simulink model "pole_cart_model"  (R2019b)
settings: Solver=VariableStepAuto  StartTime=0.0  StopTime=5  RelTol=1e-3
values from neighbouring files (symbols this model uses):
  K = zeros(Nu, Nx, Nt-1)    [run_ilqr.m]    (also in run_model.m = [ -70.7107  -37.8345  105.5298   20.9238])
  x0 = [0; 0; 0; 0]    [run_ilqr.m]    (also in run_model.m = [0;0;0;0])
settings Model: Creator=bbamin  LastModifiedBy=bbamin

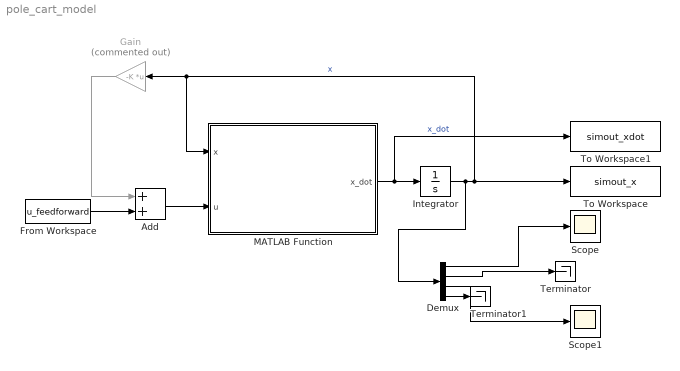
== system pole_cart_model ==
  Add : Sum
  Demux : Demux
  From Workspace : FromWorkspace  VariableName=u_feedforward  SampleTime=0  Interpolate=off  OutputAfterFinalValue=Setting to zero
  Gain : Gain  Commented=on  Gain=-K  Multiplication=Matrix(K*u)
  Integrator : Integrator  InitialCondition=x0
  MATLAB Function : MATLAB Function  TreatAsAtomicUnit=on
  Scope : Scope
  Scope1 : Scope
  Terminator : Terminator
  Terminator1 : Terminator
  To Workspace : ToWorkspace  VariableName=simout_x  SaveFormat=Timeseries  SampleTime=-1
  To Workspace1 : ToWorkspace  VariableName=simout_xdot  SaveFormat=Timeseries  SampleTime=-1
  wires:
  MATLAB Function/1(x_dot) -> To Workspace1/1, Integrator/1  "x_dot"
  Demux/1 -> Scope/1
  Demux/3 -> Scope1/1
  Integrator/1 -> MATLAB Function/1(x), Gain/1, To Workspace/1, Demux/1  "x"
  Gain/1 -> Add/1
  Add/1 -> MATLAB Function/2(u)
  From Workspace/1 -> Add/2
  Demux/2 -> Terminator/1
  Demux/4 -> Terminator1/1

== matlab function pole_cart_model/MATLAB Function ==
  data: x input; u input; x_dot output size=4
function x_dot = pole_cart_dynamics_wrapper(x, u)

x_dot = pole_cart_dynamics(x, u);
